simulink model "Bitem1"  (R2017a)
settings: Solver=VariableStepAuto  StartTime=0.0  StopTime=30  RelTol=1e-3
settings Model: Creator=julia  LastModifiedBy=julia

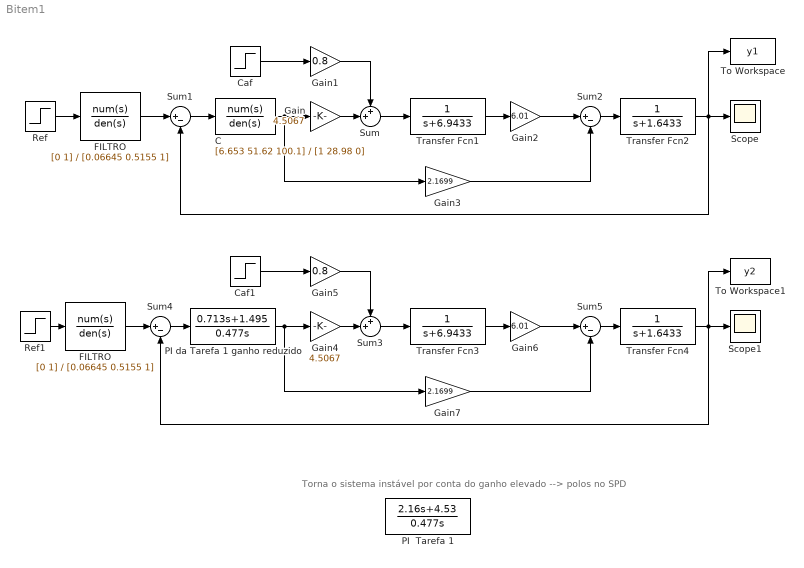
== system Bitem1 ==
  note: Torna o sistema instável por conta do ganho elevado --> polos no SPD
  C : TransferFcn  Numerator=[6.653 51.62 100.1]  Denominator=[1 28.98 0]
  Caf : Step  Time=20  SampleTime=0
  Caf1 : Step  Time=20  SampleTime=0
  "FILTRO " : TransferFcn  Numerator=[0 1]  Denominator=[0.06645 0.5155 1]
  "FILTRO  " : TransferFcn  Numerator=[0 1]  Denominator=[0.06645 0.5155 1]
  Gain : Gain  Gain=4.5067
  Gain1 : Gain  Gain=0.8
  Gain2 : Gain  Gain=6.01
  Gain3 : Gain  Gain=2.1699
  Gain4 : Gain  Gain=4.5067
  Gain5 : Gain  Gain=0.8
  Gain6 : Gain  Gain=6.01
  Gain7 : Gain  Gain=2.1699
  PI  Tarefa 1 : TransferFcn  Numerator=[2.16 4.53]  Denominator=[0.477 0]
  PI da Tarefa 1 ganho reduzido : TransferFcn  Numerator="[0.713  1.495]"  Denominator=[0.477 0]
  Ref : Step  Time=0  SampleTime=0
  Ref1 : Step  Time=0  SampleTime=0
  Scope : Scope
  Scope1 : Scope
  Sum : Sum  Inputs=++|
  Sum{1..2,4..5} (4 alike) : Sum  Inputs=|+-
  Sum3 : Sum  Inputs=++|
  To Workspace : ToWorkspace  VariableName=y1  SaveFormat=Timeseries  SampleTime=-1
  To Workspace1 : ToWorkspace  VariableName=y2  SaveFormat=Timeseries  SampleTime=-1
  Transfer Fcn1 : TransferFcn  Denominator=[1 6.9433]
  Transfer Fcn2 : TransferFcn  Denominator=[1 1.6433]
  Transfer Fcn3 : TransferFcn  Denominator=[1 6.9433]
  Transfer Fcn4 : TransferFcn  Denominator=[1 1.6433]
  wires:
  C/1 -> Gain3/1, Gain/1
  Sum1/1 -> C/1
  Gain/1 -> Sum/2
  Gain1/1 -> Sum/1
  Sum/1 -> Transfer Fcn1/1
  Transfer Fcn1/1 -> Gain2/1
  Gain2/1 -> Sum2/1
  Gain3/1 -> Sum2/2
  Sum2/1 -> Transfer Fcn2/1
  Transfer Fcn2/1 -> To Workspace/1, Sum1/2, Scope/1
  Caf/1 -> Gain1/1
  Caf1/1 -> Gain5/1
  Transfer Fcn4/1 -> To Workspace1/1, Scope1/1, Sum4/2
  Sum5/1 -> Transfer Fcn4/1
  Gain7/1 -> Sum5/2
  Gain6/1 -> Sum5/1
  Transfer Fcn3/1 -> Gain6/1
  Sum3/1 -> Transfer Fcn3/1
  Gain5/1 -> Sum3/1
  Gain4/1 -> Sum3/2
  Sum4/1 -> PI da Tarefa 1 ganho reduzido/1
  PI da Tarefa 1 ganho reduzido/1 -> Gain4/1, Gain7/1
  "FILTRO "/1 -> Sum1/1
  Ref/1 -> "FILTRO "/1
  Ref1/1 -> "FILTRO  "/1
  "FILTRO  "/1 -> Sum4/1
